simulink model "MCU_CmdTrans"  (R2022b)
settings: Solver=FixedStepDiscrete  StartTime=0.0  StopTime=10.0  FixedStep=0.001  RelTol=1e-3
undefined symbols (not defined in the file or in its folder): ANALOG, cAgeingMode, cCurrentLoopMode, cNoneMode, cParaRecogMode, cSingleBoardMode, cSpeedLoopMode, cTorqueLoopMode, cVvvfOpenMode, FAULT, ParamCfg_CommandSource_u16, ParamCfg_MaxSpeed_u16, ParamCfg_MaxTorque_u16, ParamCfg_Spdouttype_u16, ParamCfg_Vc1Enable_u16, POWER_ON, STANDBY, TESTBED, VEHICLE, WORKING
libraries: simulink x9
(part 1 of 2)
settings Model: DataDictionary=MCU_CmdTrans_Sldd_objects.sldd  Creator=ZYH  LastModifiedBy=ZYH
settings OptimizationCC: DefaultParameterBehavior=Inlined  EnhancedBackFolding=on  PassReuseOutputArgsAs=Individual arguments  OptimizeBlockOrder=speed  DifferentSizesBufferReuse=on  OptimizationCustomize=off  EfficientTunableParamExpr=on
settings DebuggingCC: ParameterTunabilityLossMsg=error
settings SFSimCC: MATLABDynamicMemAlloc=off
settings RTWCC: Description=Embedded Coder  SystemTargetFile=ert.tlc  GenCodeOnly=on  TemplateMakefile=ert_default_tmf
settings CodeAppCC: ForceParamTrailComments=on  IgnoreCustomStorageClasses=off  OperatorAnnotations=on  SimulinkDataObjDesc=on  SFDataObjDesc=on  InsertBlockDesc=on
settings ERTTargetCC: TargetLangStandard=C99 (ISO)  GenerateSampleERTMain=on  InlinedParameterPlacement=NonHierarchical  ERTCustomFileTemplate=example_file_process.tlc

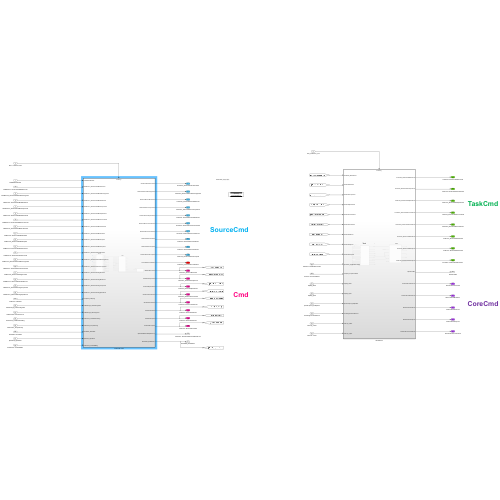
[thumbnail: Simulink's stored preview of the top-level diagram]
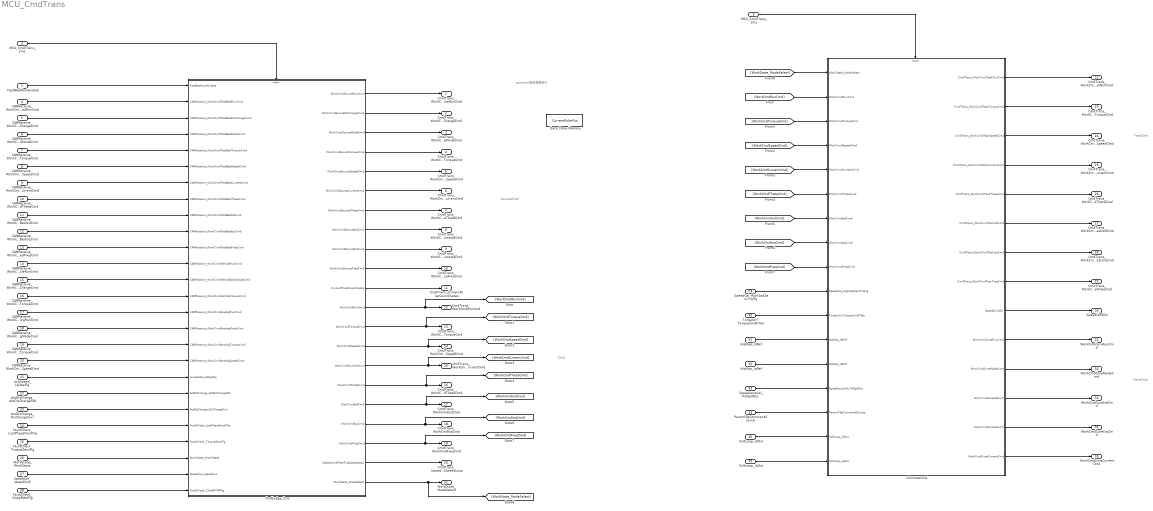
== system MCU_CmdTrans ==
  note: workcmd是否需要简化
  note: TaskCmd
  note: CoreCmd
  note: Cmd
  note: SourceCmd
  TestBedWorkEnable : Inport
  MCU_CmdTrans_1ms : Inport  Port=2  SampleTime=0.001  OutputFunctionCall=on
  MCU_CmdTrans_2ms : Inport  Port=3  SampleTime=0.002  OutputFunctionCall=on
  CANReceive_WorkCmdTestBedRunCmd : Inport  Port=4
  CANReceive_WorkCmdTestBedDisChargeCmd : Inport  Port=5
  CANReceive_WorkCmdTestBedModeCmd : Inport  Port=6
  CANReceive_WorkCmdTestBedTorqueCmd : Inport  Port=7
  CANReceive_WorkCmdTestBedSpeedCmd : Inport  Port=8
  CANReceive_WorkCmdTestBedCurrentCmd : Inport  Port=9
  CANReceive_WorkCmdTestBedThetaCmd : Inport  Port=10
  CANReceive_WorkCmdTestBedIsdCmd : Inport  Port=11
  CANReceive_WorkCmdTestBedIsqCmd : Inport  Port=12
  CANReceive_WorkCmdTestBedFreqCmd : Inport  Port=13
  CANReceive_WorkCmdVehicleRunCmd : Inport  Port=14
  CANReceive_WorkCmdVehicleDisChargeCmd : Inport  Port=15
  CANReceive_WorkCmdVehicleTorqueCmd : Inport  Port=16
  CANReceive_WorkCmdAnalogRunCmd : Inport  Port=17
  CANReceive_WorkCmdAnalogModeCmd : Inport  Port=18
  CANReceive_WorkCmdAnalogTorqueCmd : Inport  Port=19
  CANReceive_WorkCmdAnalogSpeedCmd : Inport  Port=20
  LowSpeed_LsDepFlg : Inport  Port=21
  ActDisCharge_ActDisChargeStd : Inport  Port=22
  ActDisCharge_DisChargeCurr : Inport  Port=23
  FaultCheck_LostPhaseFaultFlg : Inport  Port=24
  FaultCheck_TorqueZeroFlg : Inport  Port=25
  WorkState_WorkState : Inport  Port=26
  SpeedCal_speed2ms : Inport  Port=27
  FaultCheck_ClosePWMFlg : Inport  Port=28
  SpeedCal_HighSpdZeroTrqFlg : Inport  Port=29
  TorqeCtrl_TorqueCmdFilter : Inport  Port=30
  IdqMap_IdRef : Inport  Port=31
  IdqMap_IqRef : Inport  Port=32
  SpeedLoopCal_PidSpdOut : Inport  Port=33
  ParamCfgCommandSource : Inport  Port=34
  VoltLoop_IdOut : Inport  Port=35
  VoltLoop_IqOut : Inport  Port=36
  CmdJudge_2ms : Subsystem
  Data Store Memory : DataStoreMemory  DataStoreName=CurrentPolarFuc  WriteAfterWriteMsg=warning  ShareAcrossModelInstances=on  ShowAdditionalParam=off
  UltimateCmd : Subsystem  TreatAsAtomicUnit=on
  CmdTrans_WorkCmdSourceRunCmd : Outport
  CmdTrans_WorkCmdSourceDisChargeCmd : Outport  Port=2
  CmdTrans_WorkCmdSourceModeCmd : Outport  Port=3
  CmdTrans_WorkCmdSourceTorqueCmd : Outport  Port=4
  CmdTrans_WorkCmdSourceSpeedCmd : Outport  Port=5
  CmdTrans_WorkCmdSourceCurrentCmd : Outport  Port=6
  CmdTrans_WorkCmdSourceThetaCmd : Outport  Port=7
  CmdTrans_WorkCmdSourceIsdCmd : Outport  Port=8
  CmdTrans_WorkCmdSourceIsqCmd : Outport  Port=9
  CmdTrans_WorkCmdSourceFreqCmd : Outport  Port=10
  CmdTrans_CurrentPolarCoordinates : Outport  Port=11
  CmdTrans_WorkCmdRunCmd : Outport  Port=12
  CmdTrans_WorkCmdTorqueCmd : Outport  Port=13
  CmdTrans_WorkCmdSpeedCmd : Outport  Port=14
  CmdTrans_WorkCmdCurrentCmd : Outport  Port=15
  CmdTrans_WorkCmdThetaCmd : Outport  Port=16
  CmdTrans_WorkCmdIsdCmd : Outport  Port=17
  CmdTrans_WorkCmdIsqCmd : Outport  Port=18
  CmdTrans_WorkCmdFreqCmd : Outport  Port=19
  CmdTrans_SpeedCmdFilterFirstSpeedLoop : Outport  Port=20
  WorkState_ModeSelect : Outport  Port=21
  CmdTrans_WorkCmdTaskRunCmd : Outport  Port=22
  CmdTrans_WorkCmdTaskTorqueCmd : Outport  Port=23
  CmdTrans_WorkCmdTaskSpeedCmd : Outport  Port=24
  CmdTrans_WorkCmdTaskCurrentCmd : Outport  Port=25
  CmdTrans_WorkCmdTaskThetaCmd : Outport  Port=26
  CmdTrans_WorkCmdTaskIsdCmd : Outport  Port=27
  CmdTrans_WorkCmdTaskIsqCmd : Outport  Port=28
  CmdTrans_WorkCmdTaskFreqCmd : Outport  Port=29
  SpeedCmdDir : Outport  Port=30
  WorkCmdCoreRunCmd : Outport  Port=31
  WorkCmdCoreModeCmd : Outport  Port=32
  WorkCmdCoreIsdCmd : Outport  Port=33
  WorkCmdCoreIsqCmd : Outport  Port=34
  WorkCmdCoreCurrentCmd : Outport  Port=35
  wires:
  CANReceive_WorkCmdTestBedRunCmd/1 -> CmdJudge_2ms/2(CANReceive_WorkCmdTestBedRunCmd)
  CANReceive_WorkCmdTestBedDisChargeCmd/1 -> CmdJudge_2ms/3(CANReceive_WorkCmdTestBedDisChargeCmd)
  CANReceive_WorkCmdTestBedModeCmd/1 -> CmdJudge_2ms/4(CANReceive_WorkCmdTestBedModeCmd)
  CANReceive_WorkCmdTestBedTorqueCmd/1 -> CmdJudge_2ms/5(CANReceive_WorkCmdTestBedTorqueCmd)
  CANReceive_WorkCmdTestBedSpeedCmd/1 -> CmdJudge_2ms/6(CANReceive_WorkCmdTestBedSpeedCmd)
  CANReceive_WorkCmdTestBedCurrentCmd/1 -> CmdJudge_2ms/7(CANReceive_WorkCmdTestBedCurrentCmd)
  CANReceive_WorkCmdTestBedThetaCmd/1 -> CmdJudge_2ms/8(CANReceive_WorkCmdTestBedThetaCmd)
  CANReceive_WorkCmdTestBedIsdCmd/1 -> CmdJudge_2ms/9(CANReceive_WorkCmdTestBedIsdCmd)
  CANReceive_WorkCmdTestBedIsqCmd/1 -> CmdJudge_2ms/10(CANReceive_WorkCmdTestBedIsqCmd)
  CANReceive_WorkCmdTestBedFreqCmd/1 -> CmdJudge_2ms/11(CANReceive_WorkCmdTestBedFreqCmd)
  CANReceive_WorkCmdVehicleRunCmd/1 -> CmdJudge_2ms/12(CANReceive_WorkCmdVehicleRunCmd)
  CANReceive_WorkCmdVehicleDisChargeCmd/1 -> CmdJudge_2ms/13(CANReceive_WorkCmdVehicleDisChargeCmd)
  CANReceive_WorkCmdVehicleTorqueCmd/1 -> CmdJudge_2ms/14(CANReceive_WorkCmdVehicleTorqueCmd)
  CANReceive_WorkCmdAnalogRunCmd/1 -> CmdJudge_2ms/15(CANReceive_WorkCmdAnalogRunCmd)
  CANReceive_WorkCmdAnalogModeCmd/1 -> CmdJudge_2ms/16(CANReceive_WorkCmdAnalogModeCmd)
  CANReceive_WorkCmdAnalogTorqueCmd/1 -> CmdJudge_2ms/17(CANReceive_WorkCmdAnalogTorqueCmd)
  CANReceive_WorkCmdAnalogSpeedCmd/1 -> CmdJudge_2ms/18(CANReceive_WorkCmdAnalogSpeedCmd)
  MCU_CmdTrans_2ms/1 -> CmdJudge_2ms/Trigger
  TestBedWorkEnable/1 -> CmdJudge_2ms/1(TestBedWorkEnable)
  LowSpeed_LsDepFlg/1 -> CmdJudge_2ms/19(LowSpeed_LsDepFlg)
  ActDisCharge_ActDisChargeStd/1 -> CmdJudge_2ms/20(ActDisCharge_ActDisChargeStd)
  ActDisCharge_DisChargeCurr/1 -> CmdJudge_2ms/21(ActDisCharge_DisChargeCurr)
  FaultCheck_LostPhaseFaultFlg/1 -> CmdJudge_2ms/22(FaultCheck_LostPhaseFaultFlg)
  CmdJudge_2ms/1(WorkCmdSourceRunCmd) -> CmdTrans_WorkCmdSourceRunCmd/1
  CmdJudge_2ms/2(WorkCmdSourceDisChargeCmd) -> CmdTrans_WorkCmdSourceDisChargeCmd/1
  CmdJudge_2ms/3(WorkCmdSourceModeCmd) -> CmdTrans_WorkCmdSourceModeCmd/1
  CmdJudge_2ms/4(WorkCmdSourceTorqueCmd) -> CmdTrans_WorkCmdSourceTorqueCmd/1
  CmdJudge_2ms/5(WorkCmdSourceSpeedCmd) -> CmdTrans_WorkCmdSourceSpeedCmd/1
  CmdJudge_2ms/6(WorkCmdSourceCurrentCmd) -> CmdTrans_WorkCmdSourceCurrentCmd/1
  CmdJudge_2ms/7(WorkCmdSourceThetaCmd) -> CmdTrans_WorkCmdSourceThetaCmd/1
  CmdJudge_2ms/8(WorkCmdSourceIsdCmd) -> CmdTrans_WorkCmdSourceIsdCmd/1
  CmdJudge_2ms/9(WorkCmdSourceIsqCmd) -> CmdTrans_WorkCmdSourceIsqCmd/1
  CmdJudge_2ms/10(WorkCmdSourceFreqCmd) -> CmdTrans_WorkCmdSourceFreqCmd/1
  CmdJudge_2ms/11(CurrentPolarCoordinates) -> CmdTrans_CurrentPolarCoordinates/1
  FaultCheck_TorqueZeroFlg/1 -> CmdJudge_2ms/23(FaultCheck_TorqueZeroFlg)
  WorkState_WorkState/1 -> CmdJudge_2ms/24(WorkState_WorkState)
  SpeedCal_speed2ms/1 -> CmdJudge_2ms/25(SpeedCal_speed2ms)
  FaultCheck_ClosePWMFlg/1 -> CmdJudge_2ms/26(FaultCheck_ClosePWMFlg)
  CmdJudge_2ms/12(WorkCmdRunCmd) -> [WorkCmdRunCmd], CmdTrans_WorkCmdRunCmd/1
  CmdJudge_2ms/13(WorkCmdTorqueCmd) -> [WorkCmdTorqueCmd], CmdTrans_WorkCmdTorqueCmd/1
  CmdJudge_2ms/14(WorkCmdSpeedCmd) -> [WorkCmdSpeedCmd], CmdTrans_WorkCmdSpeedCmd/1
  CmdJudge_2ms/15(WorkCmdCurrentCmd) -> [WorkCmdCurrentCmd], CmdTrans_WorkCmdCurrentCmd/1
  CmdJudge_2ms/16(WorkCmdThetaCmd) -> [WorkCmdThetaCmd], CmdTrans_WorkCmdThetaCmd/1
  CmdJudge_2ms/17(WorkCmdIsdCmd) -> [WorkCmdIsdCmd], CmdTrans_WorkCmdIsdCmd/1
  CmdJudge_2ms/18(WorkCmdIsqCmd) -> [WorkCmdIsqCmd], CmdTrans_WorkCmdIsqCmd/1
  CmdJudge_2ms/19(WorkCmdFreqCmd) -> [WorkCmdFreqCmd], CmdTrans_WorkCmdFreqCmd/1
  CmdJudge_2ms/20(SpeedCmdFilterFirstSpeedLoop) -> CmdTrans_SpeedCmdFilterFirstSpeedLoop/1
  MCU_CmdTrans_1ms/1 -> UltimateCmd/Trigger
  CmdJudge_2ms/21(WorkState_ModeSelect) -> [WorkState_ModeSelect], WorkState_ModeSelect/1
  [WorkState_ModeSelect] -> UltimateCmd/1(WorkState_ModeSelect)
  [WorkCmdRunCmd] -> UltimateCmd/2(WorkCmdRunCmd)
  [WorkCmdTorqueCmd] -> UltimateCmd/3(WorkCmdTorqueCmd)
  [WorkCmdSpeedCmd] -> UltimateCmd/4(WorkCmdSpeedCmd)
  [WorkCmdCurrentCmd] -> UltimateCmd/5(WorkCmdCurrentCmd)
  [WorkCmdThetaCmd] -> UltimateCmd/6(WorkCmdThetaCmd)
  [WorkCmdIsdCmd] -> UltimateCmd/7(WorkCmdIsdCmd)
  [WorkCmdIsqCmd] -> UltimateCmd/8(WorkCmdIsqCmd)
  [WorkCmdFreqCmd] -> UltimateCmd/9(WorkCmdFreqCmd)
  TorqeCtrl_TorqueCmdFilter/1 -> UltimateCmd/11(TorqeCtrl_TorqueCmdFilter)
  SpeedCal_HighSpdZeroTrqFlg/1 -> UltimateCmd/10(SpeedCal_HighSpdZeroTrqFlg)
  UltimateCmd/1(CmdTrans_WorkCmdTaskRunCmd) -> CmdTrans_WorkCmdTaskRunCmd/1
  UltimateCmd/2(CmdTrans_WorkCmdTaskTorqueCmd) -> CmdTrans_WorkCmdTaskTorqueCmd/1
  UltimateCmd/3(CmdTrans_WorkCmdTaskSpeedCmd) -> CmdTrans_WorkCmdTaskSpeedCmd/1
  UltimateCmd/4(CmdTrans_WorkCmdTaskCurrentCmd) -> CmdTrans_WorkCmdTaskCurrentCmd/1
  UltimateCmd/5(CmdTrans_WorkCmdTaskThetaCmd) -> CmdTrans_WorkCmdTaskThetaCmd/1
  UltimateCmd/6(CmdTrans_WorkCmdTaskIsdCmd) -> CmdTrans_WorkCmdTaskIsdCmd/1
  UltimateCmd/7(CmdTrans_WorkCmdTaskIsqCmd) -> CmdTrans_WorkCmdTaskIsqCmd/1
  UltimateCmd/8(CmdTrans_WorkCmdTaskFreqCmd) -> CmdTrans_WorkCmdTaskFreqCmd/1
  UltimateCmd/9(SpeedCmdDir) -> SpeedCmdDir/1
  VoltLoop_IqOut/1 -> UltimateCmd/17(VoltLoop_IqOut)
  IdqMap_IdRef/1 -> UltimateCmd/12(IdqMap_IdRef)
  ParamCfgCommandSource/1 -> UltimateCmd/15(ParamCfgCommandSource)
  VoltLoop_IdOut/1 -> UltimateCmd/16(VoltLoop_IdOut)
  SpeedLoopCal_PidSpdOut/1 -> UltimateCmd/14(SpeedLoopCal_PidSpdOut)
  IdqMap_IqRef/1 -> UltimateCmd/13(IdqMap_IqRef)
  UltimateCmd/10(WorkCmdCoreRunCmd) -> WorkCmdCoreRunCmd/1
  UltimateCmd/11(WorkCmdCoreModeCmd) -> WorkCmdCoreModeCmd/1
  UltimateCmd/12(WorkCmdCoreIsdCmd) -> WorkCmdCoreIsdCmd/1
  UltimateCmd/13(WorkCmdCoreIsqCmd) -> WorkCmdCoreIsqCmd/1
  UltimateCmd/14(WorkCmdCoreCurrentCmd) -> WorkCmdCoreCurrentCmd/1

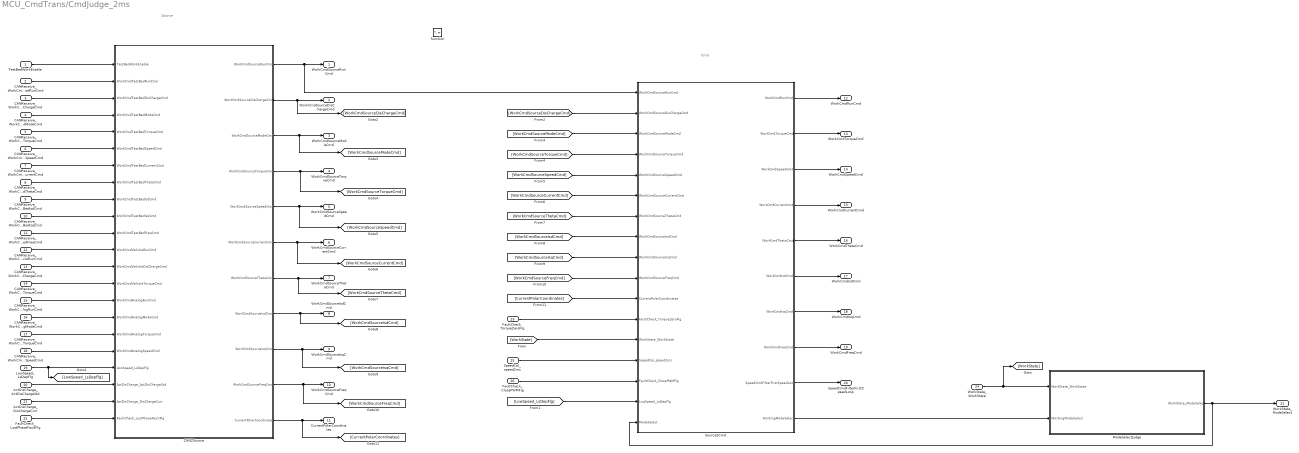
== system MCU_CmdTrans/CmdJudge_2ms ==
  note: Cmd
  note: Source
  TestBedWorkEnable : Inport
  CANReceive_WorkCmdTestBedRunCmd : Inport  Port=2
  CANReceive_WorkCmdTestBedDisChargeCmd : Inport  Port=3
  CANReceive_WorkCmdTestBedModeCmd : Inport  Port=4
  CANReceive_WorkCmdTestBedTorqueCmd : Inport  Port=5
  CANReceive_WorkCmdTestBedSpeedCmd : Inport  Port=6
  CANReceive_WorkCmdTestBedCurrentCmd : Inport  Port=7
  CANReceive_WorkCmdTestBedThetaCmd : Inport  Port=8
  CANReceive_WorkCmdTestBedIsdCmd : Inport  Port=9
  CANReceive_WorkCmdTestBedIsqCmd : Inport  Port=10
  CANReceive_WorkCmdTestBedFreqCmd : Inport  Port=11
  CANReceive_WorkCmdVehicleRunCmd : Inport  Port=12
  CANReceive_WorkCmdVehicleDisChargeCmd : Inport  Port=13
  CANReceive_WorkCmdVehicleTorqueCmd : Inport  Port=14
  CANReceive_WorkCmdAnalogRunCmd : Inport  Port=15
  CANReceive_WorkCmdAnalogModeCmd : Inport  Port=16
  CANReceive_WorkCmdAnalogTorqueCmd : Inport  Port=17
  CANReceive_WorkCmdAnalogSpeedCmd : Inport  Port=18
  LowSpeed_LsDepFlg : Inport  Port=19
  ActDisCharge_ActDisChargeStd : Inport  Port=20
  ActDisCharge_DisChargeCurr : Inport  Port=21
  FaultCheck_LostPhaseFaultFlg : Inport  Port=22
  FaultCheck_TorqueZeroFlg : Inport  Port=23
  WorkState_WorkState : Inport  Port=24
  SpeedCal_speed2ms : Inport  Port=25
  FaultCheck_ClosePWMFlg : Inport  Port=26
  function : TriggerPort  TriggerType=function-call  VariantControl=(inherit)
  CAN2Source : Subsystem  TreatAsAtomicUnit=on
      settings: RTWSystemCode=Nonreusable function
  ModeSelectJudge : Subsystem  TreatAsAtomicUnit=on
      settings: RTWSystemCode=Nonreusable function
  Source2Cmd : Subsystem  TreatAsAtomicUnit=on
      settings: RTWSystemCode=Nonreusable function
  WorkCmdSourceRunCmd : Outport
  WorkCmdSourceDisChargeCmd : Outport  Port=2
  WorkCmdSourceModeCmd : Outport  Port=3
  WorkCmdSourceTorqueCmd : Outport  Port=4
  WorkCmdSourceSpeedCmd : Outport  Port=5
  WorkCmdSourceCurrentCmd : Outport  Port=6
  WorkCmdSourceThetaCmd : Outport  Port=7
  WorkCmdSourceIsdCmd : Outport  Port=8
  WorkCmdSourceIsqCmd : Outport  Port=9
  WorkCmdSourceFreqCmd : Outport  Port=10
  CurrentPolarCoordinates : Outport  Port=11
  WorkCmdRunCmd : Outport  Port=12
  WorkCmdTorqueCmd : Outport  Port=13
  WorkCmdSpeedCmd : Outport  Port=14
  WorkCmdCurrentCmd : Outport  Port=15
  WorkCmdThetaCmd : Outport  Port=16
  WorkCmdIsdCmd : Outport  Port=17
  WorkCmdIsqCmd : Outport  Port=18
  WorkCmdFreqCmd : Outport  Port=19
  SpeedCmdFilterFirstSpeedLoop : Outport  Port=20
  WorkState_ModeSelect : Outport  Port=21
  wires:
  CANReceive_WorkCmdVehicleTorqueCmd/1 -> CAN2Source/14(WorkCmdVehicleTorqueCmd)
  CANReceive_WorkCmdTestBedSpeedCmd/1 -> CAN2Source/6(WorkCmdTestBedSpeedCmd)
  CANReceive_WorkCmdTestBedIsqCmd/1 -> CAN2Source/10(WorkCmdTestBedIsqCmd)
  CANReceive_WorkCmdAnalogModeCmd/1 -> CAN2Source/16(WorkCmdAnalogModeCmd)
  CANReceive_WorkCmdTestBedTorqueCmd/1 -> CAN2Source/5(WorkCmdTestBedTorqueCmd)
  CANReceive_WorkCmdTestBedRunCmd/1 -> CAN2Source/2(WorkCmdTestBedRunCmd)
  CANReceive_WorkCmdTestBedFreqCmd/1 -> CAN2Source/11(WorkCmdTestBedFreqCmd)
  CANReceive_WorkCmdTestBedIsdCmd/1 -> CAN2Source/9(WorkCmdTestBedIsdCmd)
  CANReceive_WorkCmdAnalogRunCmd/1 -> CAN2Source/15(WorkCmdAnalogRunCmd)
  CANReceive_WorkCmdAnalogTorqueCmd/1 -> CAN2Source/17(WorkCmdAnalogTorqueCmd)
  CANReceive_WorkCmdTestBedCurrentCmd/1 -> CAN2Source/7(WorkCmdTestBedCurrentCmd)
  CANReceive_WorkCmdTestBedDisChargeCmd/1 -> CAN2Source/3(WorkCmdTestBedDisChargeCmd)
  CANReceive_WorkCmdVehicleDisChargeCmd/1 -> CAN2Source/13(WorkCmdVehicleDisChargeCmd)
  CANReceive_WorkCmdAnalogSpeedCmd/1 -> CAN2Source/18(WorkCmdAnalogSpeedCmd)
  CANReceive_WorkCmdTestBedThetaCmd/1 -> CAN2Source/8(WorkCmdTestBedThetaCmd)
  CANReceive_WorkCmdTestBedModeCmd/1 -> CAN2Source/4(WorkCmdTestBedModeCmd)
  CANReceive_WorkCmdVehicleRunCmd/1 -> CAN2Source/12(WorkCmdVehicleRunCmd)
  TestBedWorkEnable/1 -> CAN2Source/1(TestBedWorkEnable)
  CAN2Source/11(CurrentPolarCoordinates) -> [CurrentPolarCoordinates], CurrentPolarCoordinates/1
  CAN2Source/2(WorkCmdSourceDisChargeCmd) -> [WorkCmdSourceDisChargeCmd], WorkCmdSourceDisChargeCmd/1
  CAN2Source/3(WorkCmdSourceModeCmd) -> [WorkCmdSourceModeCmd], WorkCmdSourceModeCmd/1
  CAN2Source/4(WorkCmdSourceTorqueCmd) -> [WorkCmdSourceTorqueCmd], WorkCmdSourceTorqueCmd/1
  CAN2Source/5(WorkCmdSourceSpeedCmd) -> [WorkCmdSourceSpeedCmd], WorkCmdSourceSpeedCmd/1
  CAN2Source/6(WorkCmdSourceCurrentCmd) -> [WorkCmdSourceCurrentCmd], WorkCmdSourceCurrentCmd/1
  CAN2Source/7(WorkCmdSourceThetaCmd) -> [WorkCmdSourceThetaCmd], WorkCmdSourceThetaCmd/1
  CAN2Source/8(WorkCmdSourceIsdCmd) -> [WorkCmdSourceIsdCmd], WorkCmdSourceIsdCmd/1
  CAN2Source/9(WorkCmdSourceIsqCmd) -> [WorkCmdSourceIsqCmd], WorkCmdSourceIsqCmd/1
  CAN2Source/10(WorkCmdSourceFreqCmd) -> WorkCmdSourceFreqCmd/1, [WorkCmdSourceFreqCmd]
  LowSpeed_LsDepFlg/1 -> [LowSpeed_LsDepFlg], CAN2Source/19(LowSpeed_LsDepFlg)
  ActDisCharge_DisChargeCurr/1 -> CAN2Source/21(ActDisCharge_DisChargeCurr)
  FaultCheck_LostPhaseFaultFlg/1 -> CAN2Source/22(FaultCheck_LostPhaseFaultFlg)
  ActDisCharge_ActDisChargeStd/1 -> CAN2Source/20(ActDisCharge_ActDisChargeStd)
  ModeSelectJudge/1(WorkState_ModeSelect) -> WorkState_ModeSelect/1, Source2Cmd/17(ModeSelect)
  FaultCheck_TorqueZeroFlg/1 -> Source2Cmd/12(FaultCheck_TorqueZeroFlg)
  SpeedCal_speed2ms/1 -> Source2Cmd/14(SpeedCal_speed2ms)
  WorkState_WorkState/1 -> [WorkState], ModeSelectJudge/1(WorkState_WorkState)
  FaultCheck_ClosePWMFlg/1 -> Source2Cmd/15(FaultCheck_ClosePWMFlg)
  Source2Cmd/1(WorkCmdRunCmd) -> WorkCmdRunCmd/1
  Source2Cmd/2(WorkCmdTorqueCmd) -> WorkCmdTorqueCmd/1
  Source2Cmd/3(WorkCmdSpeedCmd) -> WorkCmdSpeedCmd/1
  Source2Cmd/4(WorkCmdCurrentCmd) -> WorkCmdCurrentCmd/1
  Source2Cmd/5(WorkCmdThetaCmd) -> WorkCmdThetaCmd/1
  Source2Cmd/6(WorkCmdIsdCmd) -> WorkCmdIsdCmd/1
  Source2Cmd/7(WorkCmdIsqCmd) -> WorkCmdIsqCmd/1
  Source2Cmd/8(WorkCmdFreqCmd) -> WorkCmdFreqCmd/1
  Source2Cmd/9(SpeedCmdFilterFirstSpeedLoop) -> SpeedCmdFilterFirstSpeedLoop/1
  CAN2Source/1(WorkCmdSourceRunCmd) -> Source2Cmd/1(WorkCmdSourceRunCmd), WorkCmdSourceRunCmd/1
  [WorkCmdSourceDisChargeCmd] -> Source2Cmd/2(WorkCmdSourceDisChargeCmd)
  [WorkCmdSourceFreqCmd] -> Source2Cmd/10(WorkCmdSourceFreqCmd)
  [WorkCmdSourceModeCmd] -> Source2Cmd/3(WorkCmdSourceModeCmd)
  [WorkCmdSourceTorqueCmd] -> Source2Cmd/4(WorkCmdSourceTorqueCmd)
  [WorkCmdSourceSpeedCmd] -> Source2Cmd/5(WorkCmdSourceSpeedCmd)
  [WorkCmdSourceCurrentCmd] -> Source2Cmd/6(WorkCmdSourceCurrentCmd)
  [WorkCmdSourceThetaCmd] -> Source2Cmd/7(WorkCmdSourceThetaCmd)
  [WorkCmdSourceIsdCmd] -> Source2Cmd/8(WorkCmdSourceIsdCmd)
  [WorkCmdSourceIsqCmd] -> Source2Cmd/9(WorkCmdSourceIsqCmd)
  [CurrentPolarCoordinates] -> Source2Cmd/11(CurrentPolarCoordinates)
  [WorkState] -> Source2Cmd/13(WorkState_WorkState)
  Source2Cmd/10(WorkingModeSelect) -> ModeSelectJudge/2(WorkingModeSelect)
  [LowSpeed_LsDepFlg] -> Source2Cmd/16(LowSpeed_LsDepFlg)

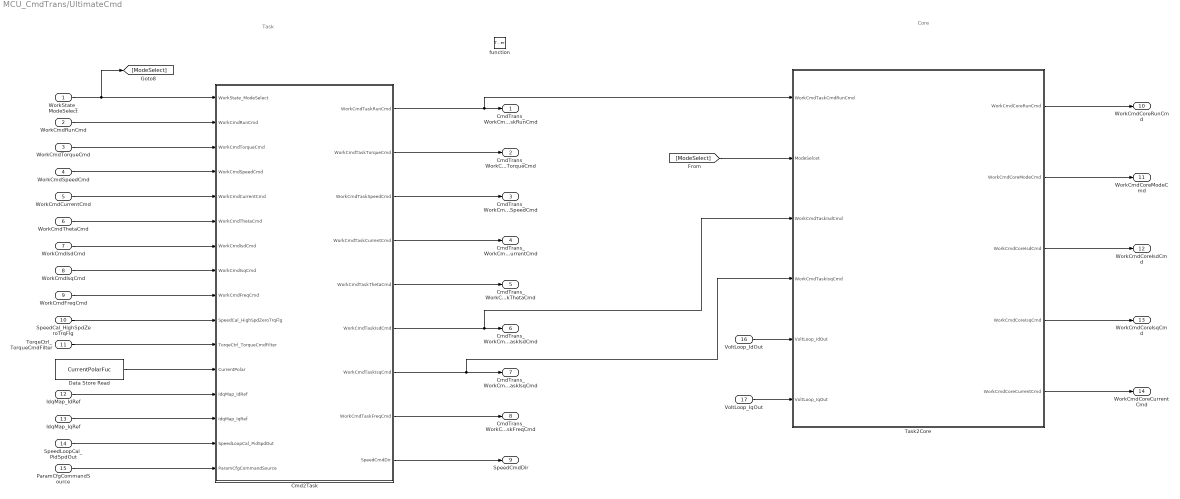
== system MCU_CmdTrans/UltimateCmd ==
  note: Core
  note: Task
  WorkState_ModeSelect : Inport
  WorkCmdRunCmd : Inport  Port=2
  WorkCmdTorqueCmd : Inport  Port=3
  WorkCmdSpeedCmd : Inport  Port=4
  WorkCmdCurrentCmd : Inport  Port=5
  WorkCmdThetaCmd : Inport  Port=6
  WorkCmdIsdCmd : Inport  Port=7
  WorkCmdIsqCmd : Inport  Port=8
  WorkCmdFreqCmd : Inport  Port=9
  SpeedCal_HighSpdZeroTrqFlg : Inport  Port=10
  TorqeCtrl_TorqueCmdFilter : Inport  Port=11
  IdqMap_IdRef : Inport  Port=12
  IdqMap_IqRef : Inport  Port=13
  SpeedLoopCal_PidSpdOut : Inport  Port=14
  ParamCfgCommandSource : Inport  Port=15
  VoltLoop_IdOut : Inport  Port=16
  VoltLoop_IqOut : Inport  Port=17
  function : TriggerPort  TriggerType=function-call  VariantControl=(inherit)
  Cmd2Task : Subsystem
  Data Store Read : DataStoreRead  DataStoreName=CurrentPolarFuc  IndexOptions=Index vector (dialog)  Indices=1  OutputSizes=1
  Task2Core : Subsystem
  CmdTrans_WorkCmdTaskRunCmd : Outport
  CmdTrans_WorkCmdTaskTorqueCmd : Outport  Port=2
  CmdTrans_WorkCmdTaskSpeedCmd : Outport  Port=3
  CmdTrans_WorkCmdTaskCurrentCmd : Outport  Port=4
  CmdTrans_WorkCmdTaskThetaCmd : Outport  Port=5
  CmdTrans_WorkCmdTaskIsdCmd : Outport  Port=6
  CmdTrans_WorkCmdTaskIsqCmd : Outport  Port=7
  CmdTrans_WorkCmdTaskFreqCmd : Outport  Port=8
  SpeedCmdDir : Outport  Port=9
  WorkCmdCoreRunCmd : Outport  Port=10
  WorkCmdCoreModeCmd : Outport  Port=11
  WorkCmdCoreIsdCmd : Outport  Port=12
  WorkCmdCoreIsqCmd : Outport  Port=13
  WorkCmdCoreCurrentCmd : Outport  Port=14
  wires:
  WorkState_ModeSelect/1 -> [ModeSelect], Cmd2Task/1(WorkState_ModeSelect)
  WorkCmdRunCmd/1 -> Cmd2Task/2(WorkCmdRunCmd)
  WorkCmdTorqueCmd/1 -> Cmd2Task/3(WorkCmdTorqueCmd)
  WorkCmdSpeedCmd/1 -> Cmd2Task/4(WorkCmdSpeedCmd)
  WorkCmdCurrentCmd/1 -> Cmd2Task/5(WorkCmdCurrentCmd)
  WorkCmdThetaCmd/1 -> Cmd2Task/6(WorkCmdThetaCmd)
  WorkCmdIsdCmd/1 -> Cmd2Task/7(WorkCmdIsdCmd)
  WorkCmdIsqCmd/1 -> Cmd2Task/8(WorkCmdIsqCmd)
  WorkCmdFreqCmd/1 -> Cmd2Task/9(WorkCmdFreqCmd)
  SpeedCal_HighSpdZeroTrqFlg/1 -> Cmd2Task/10(SpeedCal_HighSpdZeroTrqFlg)
  TorqeCtrl_TorqueCmdFilter/1 -> Cmd2Task/11(TorqeCtrl_TorqueCmdFilter)
  Data Store Read/1 -> Cmd2Task/12(CurrentPolar)
  Cmd2Task/1(WorkCmdTaskRunCmd) -> Task2Core/1(WorkCmdTaskCmdRunCmd), CmdTrans_WorkCmdTaskRunCmd/1
  Cmd2Task/2(WorkCmdTaskTorqueCmd) -> CmdTrans_WorkCmdTaskTorqueCmd/1
  Cmd2Task/3(WorkCmdTaskSpeedCmd) -> CmdTrans_WorkCmdTaskSpeedCmd/1
  Cmd2Task/4(WorkCmdTaskCurrentCmd) -> CmdTrans_WorkCmdTaskCurrentCmd/1
  Cmd2Task/5(WorkCmdTaskThetaCmd) -> CmdTrans_WorkCmdTaskThetaCmd/1
  Cmd2Task/7(WorkCmdTaskIsqCmd) -> Task2Core/4(WorkCmdTaskIsqCmd), CmdTrans_WorkCmdTaskIsqCmd/1
  Cmd2Task/8(WorkCmdTaskFreqCmd) -> CmdTrans_WorkCmdTaskFreqCmd/1
  Cmd2Task/9(SpeedCmdDir) -> SpeedCmdDir/1
  [ModeSelect] -> Task2Core/2(ModeSelcet)
  IdqMap_IqRef/1 -> Cmd2Task/14(IdqMap_IqRef)
  SpeedLoopCal_PidSpdOut/1 -> Cmd2Task/15(SpeedLoopCal_PidSpdOut)
  IdqMap_IdRef/1 -> Cmd2Task/13(IdqMap_IdRef)
  ParamCfgCommandSource/1 -> Cmd2Task/16(ParamCfgCommandSource)
  Cmd2Task/6(WorkCmdTaskIsdCmd) -> Task2Core/3(WorkCmdTaskIsdCmd), CmdTrans_WorkCmdTaskIsdCmd/1
  VoltLoop_IdOut/1 -> Task2Core/5(VoltLoop_IdOut)
  VoltLoop_IqOut/1 -> Task2Core/6(VoltLoop_IqOut)
  Task2Core/1(WorkCmdCoreRunCmd) -> WorkCmdCoreRunCmd/1
  Task2Core/3(WorkCmdCoreIsdCmd) -> WorkCmdCoreIsdCmd/1
  Task2Core/2(WorkCmdCoreModeCmd) -> WorkCmdCoreModeCmd/1
  Task2Core/4(WorkCmdCoreIsqCmd) -> WorkCmdCoreIsqCmd/1
  Task2Core/5(WorkCmdCoreCurrentCmd) -> WorkCmdCoreCurrentCmd/1

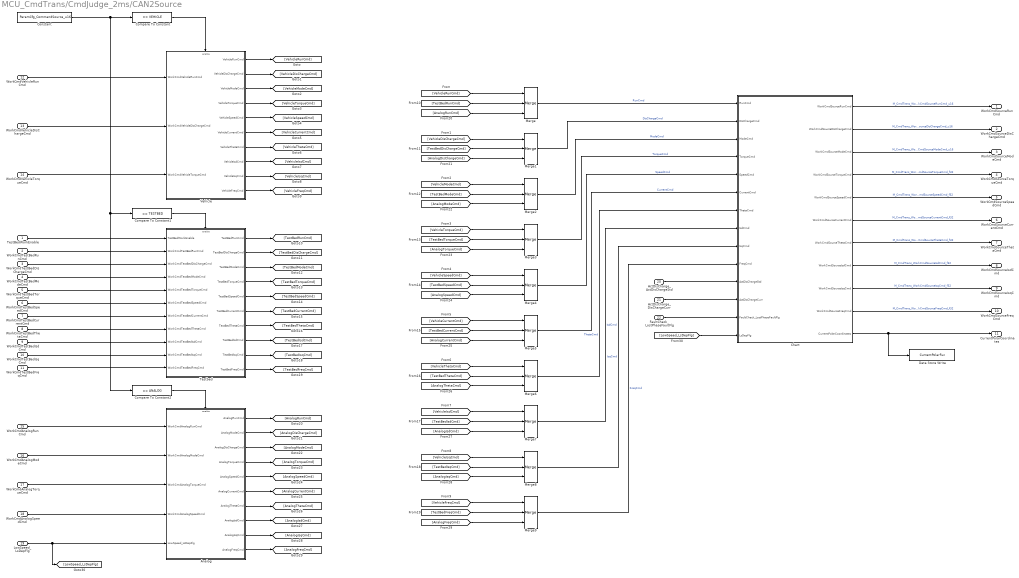
== system MCU_CmdTrans/CmdJudge_2ms/CAN2Source ==
  TestBedWorkEnable : Inport
  WorkCmdTestBedRunCmd : Inport  Port=2
  WorkCmdTestBedDisChargeCmd : Inport  Port=3
  WorkCmdTestBedModeCmd : Inport  Port=4
  WorkCmdTestBedTorqueCmd : Inport  Port=5
  WorkCmdTestBedSpeedCmd : Inport  Port=6
  WorkCmdTestBedCurrentCmd : Inport  Port=7
  WorkCmdTestBedThetaCmd : Inport  Port=8
  WorkCmdTestBedIsdCmd : Inport  Port=9
  WorkCmdTestBedIsqCmd : Inport  Port=10
  WorkCmdTestBedFreqCmd : Inport  Port=11
  WorkCmdVehicleRunCmd : Inport  Port=12
  WorkCmdVehicleDisChargeCmd : Inport  Port=13
  WorkCmdVehicleTorqueCmd : Inport  Port=14
  WorkCmdAnalogRunCmd : Inport  Port=15
  WorkCmdAnalogModeCmd : Inport  Port=16
  WorkCmdAnalogTorqueCmd : Inport  Port=17
  WorkCmdAnalogSpeedCmd : Inport  Port=18
  LowSpeed_LsDepFlg : Inport  Port=19
  ActDisCharge_ActDisChargeStd : Inport  Port=20
  ActDisCharge_DisChargeCurr : Inport  Port=21
  FaultCheck_LostPhaseFaultFlg : Inport  Port=22
  Analog : Subsystem  TreatAsAtomicUnit=on
  Chart : Stateflow chart  TreatAsAtomicUnit=on
  Compare To Constant : simulink/Logic and Bit Operations/Compare To Constant  relop===  const=VEHICLE  OutDataTypeStr=boolean
  Compare To Constant1 : simulink/Logic and Bit Operations/Compare To Constant  relop===  const=TESTBED  OutDataTypeStr=boolean
  Compare To Constant2 : simulink/Logic and Bit Operations/Compare To Constant  relop===  const=ANALOG  OutDataTypeStr=boolean
  Constant : Constant  Value=ParamCfg_CommandSource_u16
  Data Store Write : DataStoreWrite  DataStoreName=CurrentPolarFuc  IndexOptions=Index vector (dialog)  Indices=1  OutputSizes=1
  Merge{,1..9} (10 alike) : Merge  Inputs=3
  Testbed : Subsystem  TreatAsAtomicUnit=on
  Vehicle : Subsystem
  WorkCmdSourceRunCmd : Outport
  WorkCmdSourceDisChargeCmd : Outport  Port=2
  WorkCmdSourceModeCmd : Outport  Port=3
  WorkCmdSourceTorqueCmd : Outport  Port=4
  WorkCmdSourceSpeedCmd : Outport  Port=5
  WorkCmdSourceCurrentCmd : Outport  Port=6
  WorkCmdSourceThetaCmd : Outport  Port=7
  WorkCmdSourceIsdCmd : Outport  Port=8
  WorkCmdSourceIsqCmd : Outport  Port=9
  WorkCmdSourceFreqCmd : Outport  Port=10
  CurrentPolarCoordinates : Outport  Port=11
  wires:
  Constant/1 -> Compare To Constant2/1, Compare To Constant1/1, Compare To Constant/1
  Compare To Constant/1 -> Vehicle/Enable
  WorkCmdVehicleRunCmd/1 -> Vehicle/1(WorkCmdVehicleRunCmd)
  WorkCmdVehicleDisChargeCmd/1 -> Vehicle/2(WorkCmdVehicleDisChargeCmd)
  WorkCmdVehicleTorqueCmd/1 -> Vehicle/3(WorkCmdVehicleTorqueCmd)
  Compare To Constant1/1 -> Testbed/Enable
  WorkCmdTestBedModeCmd/1 -> Testbed/4(WorkCmdTestBedModeCmd)
  WorkCmdTestBedTorqueCmd/1 -> Testbed/5(WorkCmdTestBedTorqueCmd)
  WorkCmdTestBedDisChargeCmd/1 -> Testbed/3(WorkCmdTestBedDisChargeCmd)
  WorkCmdTestBedSpeedCmd/1 -> Testbed/6(WorkCmdTestBedSpeedCmd)
  WorkCmdTestBedRunCmd/1 -> Testbed/2(WorkCmdTestBedRunCmd)
  WorkCmdTestBedCurrentCmd/1 -> Testbed/7(WorkCmdTestBedCurrentCmd)
  WorkCmdTestBedThetaCmd/1 -> Testbed/8(WorkCmdTestBedThetaCmd)
  WorkCmdTestBedIsdCmd/1 -> Testbed/9(WorkCmdTestBedIsdCmd)
  WorkCmdTestBedIsqCmd/1 -> Testbed/10(WorkCmdTestBedIsqCmd)
  WorkCmdTestBedFreqCmd/1 -> Testbed/11(WorkCmdTestBedFreqCmd)
  Compare To Constant2/1 -> Analog/Enable
  WorkCmdAnalogRunCmd/1 -> Analog/1(WorkCmdAnalogRunCmd)
  WorkCmdAnalogModeCmd/1 -> Analog/2(WorkCmdAnalogModeCmd)
  WorkCmdAnalogTorqueCmd/1 -> Analog/3(WorkCmdAnalogTorqueCmd)
  WorkCmdAnalogSpeedCmd/1 -> Analog/4(WorkCmdAnalogSpeedCmd)
  TestBedWorkEnable/1 -> Testbed/1(TestBedWorkEnable)
  Vehicle/1(VehicleRunCmd) -> [VehicleRunCmd]
  Vehicle/2(VehicleDisChargeCmd) -> [VehicleDisChargeCmd]
  Vehicle/3(VehicleModeCmd) -> [VehicleModeCmd]
  Vehicle/4(VehicleTorqueCmd) -> [VehicleTorqueCmd]
  Vehicle/5(VehicleSpeedCmd) -> [VehicleSpeedCmd]
  Vehicle/6(VehicleCurrentCmd) -> [VehicleCurrentCmd]
  Vehicle/7(VehicleThetaCmd) -> [VehicleThetaCmd]
  Vehicle/8(VehicleIsdCmd) -> [VehicleIsdCmd]
  Vehicle/9(VehicleIsqCmd) -> [VehicleIsqCmd]
  Vehicle/10(VehicleFreqCmd) -> [VehicleFreqCmd]
  Testbed/2(TestBedDisChargeCmd) -> [TestBedDisChargeCmd]
  Testbed/3(TestBedModeCmd) -> [TestBedModeCmd]
  Testbed/4(TestBedTorqueCmd) -> [TestBedTorqueCmd]
  Testbed/5(TestBedSpeedCmd) -> [TestBedSpeedCmd]
  Testbed/6(TestBedCurrentCmd) -> [TestBedCurrentCmd]
  Testbed/7(TestBedThetaCmd) -> [TestBedThetaCmd]
  Testbed/8(TestBedIsdCmd) -> [TestBedIsdCmd]
  Testbed/9(TestBedIsqCmd) -> [TestBedIsqCmd]
  Testbed/10(TestBedFreqCmd) -> [TestBedFreqCmd]
  Testbed/1(TestBedRunCmd) -> [TestBedRunCmd]
  Analog/2(AnalogModeCmd) -> [AnalogDisChargeCmd]
  Analog/3(AnalogDisChargeCmd) -> [AnalogModeCmd]
  Analog/4(AnalogTorqueCmd) -> [AnalogTorqueCmd]
  Analog/5(AnalogSpeedCmd) -> [AnalogSpeedCmd]
  Analog/6(AnalogCurrentCmd) -> [AnalogCurrentCmd]
  Analog/7(AnalogThetaCmd) -> [AnalogThetaCmd]
  Analog/8(AnalogIsdCmd) -> [AnalogIsdCmd]
  Analog/9(AnalogIsqCmd) -> [AnalogIsqCmd]
  Analog/10(AnalogFreqCmd) -> [AnalogFreqCmd]
  Analog/1(AnalogRunCmd) -> [AnalogRunCmd]
  [VehicleRunCmd] -> Merge/1
  [VehicleDisChargeCmd] -> Merge1/1
  [VehicleModeCmd] -> Merge2/1
  [VehicleTorqueCmd] -> Merge3/1
  [VehicleSpeedCmd] -> Merge4/1
  [VehicleFreqCmd] -> Merge9/1
  [VehicleCurrentCmd] -> Merge5/1
  [VehicleThetaCmd] -> Merge6/1
  [VehicleIsdCmd] -> Merge7/1
  [VehicleIsqCmd] -> Merge8/1
  [TestBedRunCmd] -> Merge/2
  [TestBedDisChargeCmd] -> Merge1/2
  [TestBedModeCmd] -> Merge2/2
  [TestBedTorqueCmd] -> Merge3/2
  [TestBedSpeedCmd] -> Merge4/2
  [TestBedCurrentCmd] -> Merge5/2
  [TestBedThetaCmd] -> Merge6/2
  [TestBedIsdCmd] -> Merge7/2
  [TestBedIsqCmd] -> Merge8/2
  [TestBedFreqCmd] -> Merge9/2
  [AnalogFreqCmd] -> Merge9/3
  [AnalogRunCmd] -> Merge/3
  [AnalogDisChargeCmd] -> Merge1/3
  [AnalogModeCmd] -> Merge2/3
  [AnalogTorqueCmd] -> Merge3/3
  [AnalogSpeedCmd] -> Merge4/3
  [AnalogCurrentCmd] -> Merge5/3
  [AnalogThetaCmd] -> Merge6/3
  [AnalogIsdCmd] -> Merge7/3
  [AnalogIsqCmd] -> Merge8/3
  Merge/1 -> Chart/1(RunCmd)  "RunCmd"
  Merge1/1 -> Chart/2(DisChargeCmd)  "DisChargeCmd"
  Merge2/1 -> Chart/3(ModeCmd)  "ModeCmd"
  Merge3/1 -> Chart/4(TorqueCmd)  "TorqueCmd"
  Merge4/1 -> Chart/5(SpeedCmd)  "SpeedCmd"
  Merge5/1 -> Chart/6(CurrentCmd)  "CurrentCmd"
  Merge6/1 -> Chart/7(ThetaCmd)  "ThetaCmd"
  Merge7/1 -> Chart/8(IsdCmd)  "IsdCmd"
  Merge8/1 -> Chart/9(IsqCmd)  "IsqCmd"
  Merge9/1 -> Chart/10(FreqCmd)  "FreqCmd"
  LowSpeed_LsDepFlg/1 -> [LowSpeed_LsDepFlg], Analog/5(LowSpeed_LsDepFlg)
  Chart/1(WorkCmdSourceRunCmd) -> WorkCmdSourceRunCmd/1  "M_CmdTrans_WorkCmdSourceRunCmd_u16"
  Chart/2(WorkCmdSourceDisChargeCmd) -> WorkCmdSourceDisChargeCmd/1  "M_CmdTrans_WorkCmdSourceDisChargeCmd_u16"
  Chart/3(WorkCmdSourceModeCmd) -> WorkCmdSourceModeCmd/1  "M_CmdTrans_WorkCmdSourceModeCmd_u16"
  Chart/4(WorkCmdSourceTorqueCmd) -> WorkCmdSourceTorqueCmd/1  "M_CmdTrans_WorkCmdSourceTorqueCmd_f32"
  Chart/5(WorkCmdSourceSpeedCmd) -> WorkCmdSourceSpeedCmd/1  "M_CmdTrans_WorkCmdSourceSpeedCmd_f32"
  Chart/6(WorkCmdSourceCurrentCmd) -> WorkCmdSourceCurrentCmd/1  "M_CmdTrans_WorkCmdSourceCurrentCmd_f32"
  Chart/7(WorkCmdSourceThetaCmd) -> WorkCmdSourceThetaCmd/1  "M_CmdTrans_WorkCmdSourceThetaCmd_f32"
  Chart/8(WorkCmdSourceIsdCmd) -> WorkCmdSourceIsdCmd/1  "M_CmdTrans_WorkCmdSourceIsdCmd_f32"
  Chart/9(WorkCmdSourceIsqCmd) -> WorkCmdSourceIsqCmd/1  "M_CmdTrans_WorkCmdSourceIsqCmd_f32"
  Chart/10(WorkCmdSourceFreqCmd) -> WorkCmdSourceFreqCmd/1  "M_CmdTrans_WorkCmdSourceFreqCmd_f32"
  ActDisCharge_ActDisChargeStd/1 -> Chart/11(ActDisChargeStd)
  ActDisCharge_DisChargeCurr/1 -> Chart/12(ActDisChargeCurr)
  FaultCheck_LostPhaseFaultFlg/1 -> Chart/13(FaultCheck_LostPhaseFaultFlg)
  [LowSpeed_LsDepFlg] -> Chart/14(LsDepFlg)
  Chart/11(CurrentPolarCoordinates) -> Data Store Write/1, CurrentPolarCoordinates/1

== system MCU_CmdTrans/CmdJudge_2ms/ModeSelectJudge ==
  WorkState_WorkState : Inport
  WorkingModeSelect : Inport  Port=2
  Compare To Constant : simulink/Logic and Bit Operations/Compare To Constant  relop===  const=FAULT  OutDataTypeStr=boolean
  Compare To Constant1 : simulink/Logic and Bit Operations/Compare To Constant  relop===  const=POWER_ON  OutDataTypeStr=boolean
  Compare To Constant2 : simulink/Logic and Bit Operations/Compare To Constant  relop===  const=STANDBY  OutDataTypeStr=boolean
  Constant1 : Constant  Value=cNoneMode  VectorParams1D=off  OutDataTypeStr=uint16
  Logical Operator : Logic  Operator=OR  Inputs=3  AllPortsSameDT=off  OutDataTypeStr=boolean
  Switch : Switch  Criteria=u2 ~= 0  SaturateOnIntegerOverflow=off  InputSameDT=off
  WorkState_ModeSelect : Outport
  wires:
  Constant1/1 -> Switch/1
  Compare To Constant/1 -> Logical Operator/1
  Logical Operator/1 -> Switch/2
  WorkState_WorkState/1 -> Compare To Constant2/1, Compare To Constant1/1, Compare To Constant/1
  Compare To Constant2/1 -> Logical Operator/3
  Compare To Constant1/1 -> Logical Operator/2
  WorkingModeSelect/1 -> Switch/3
  Switch/1 -> WorkState_ModeSelect/1

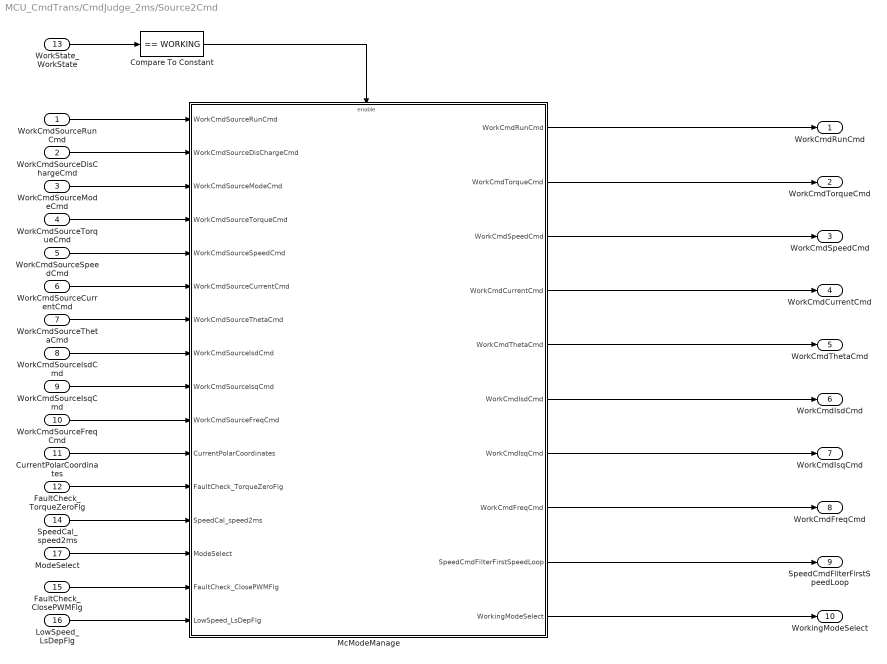
== system MCU_CmdTrans/CmdJudge_2ms/Source2Cmd ==
  WorkCmdSourceRunCmd : Inport
  WorkCmdSourceDisChargeCmd : Inport  Port=2
  WorkCmdSourceModeCmd : Inport  Port=3
  WorkCmdSourceTorqueCmd : Inport  Port=4
  WorkCmdSourceSpeedCmd : Inport  Port=5
  WorkCmdSourceCurrentCmd : Inport  Port=6
  WorkCmdSourceThetaCmd : Inport  Port=7
  WorkCmdSourceIsdCmd : Inport  Port=8
  WorkCmdSourceIsqCmd : Inport  Port=9
  WorkCmdSourceFreqCmd : Inport  Port=10
  CurrentPolarCoordinates : Inport  Port=11
  FaultCheck_TorqueZeroFlg : Inport  Port=12
  WorkState_WorkState : Inport  Port=13
  SpeedCal_speed2ms : Inport  Port=14
  FaultCheck_ClosePWMFlg : Inport  Port=15
  LowSpeed_LsDepFlg : Inport  Port=16
  ModeSelect : Inport  Port=17
  Compare To Constant : simulink/Logic and Bit Operations/Compare To Constant  relop===  const=WORKING  OutDataTypeStr=boolean
  McModeManage : Subsystem  TreatAsAtomicUnit=on
  WorkCmdRunCmd : Outport
  WorkCmdTorqueCmd : Outport  Port=2
  WorkCmdSpeedCmd : Outport  Port=3
  WorkCmdCurrentCmd : Outport  Port=4
  WorkCmdThetaCmd : Outport  Port=5
  WorkCmdIsdCmd : Outport  Port=6
  WorkCmdIsqCmd : Outport  Port=7
  WorkCmdFreqCmd : Outport  Port=8
  SpeedCmdFilterFirstSpeedLoop : Outport  Port=9
  WorkingModeSelect : Outport  Port=10
  wires:
  WorkState_WorkState/1 -> Compare To Constant/1
  Compare To Constant/1 -> McModeManage/Enable
  WorkCmdSourceDisChargeCmd/1 -> McModeManage/2(WorkCmdSourceDisChargeCmd)
  WorkCmdSourceRunCmd/1 -> McModeManage/1(WorkCmdSourceRunCmd)
  WorkCmdSourceModeCmd/1 -> McModeManage/3(WorkCmdSourceModeCmd)
  WorkCmdSourceTorqueCmd/1 -> McModeManage/4(WorkCmdSourceTorqueCmd)
  WorkCmdSourceSpeedCmd/1 -> McModeManage/5(WorkCmdSourceSpeedCmd)
  WorkCmdSourceCurrentCmd/1 -> McModeManage/6(WorkCmdSourceCurrentCmd)
  WorkCmdSourceThetaCmd/1 -> McModeManage/7(WorkCmdSourceThetaCmd)
  WorkCmdSourceIsdCmd/1 -> McModeManage/8(WorkCmdSourceIsdCmd)
  WorkCmdSourceIsqCmd/1 -> McModeManage/9(WorkCmdSourceIsqCmd)
  WorkCmdSourceFreqCmd/1 -> McModeManage/10(WorkCmdSourceFreqCmd)
  CurrentPolarCoordinates/1 -> McModeManage/11(CurrentPolarCoordinates)
  ModeSelect/1 -> McModeManage/14(ModeSelect)
  FaultCheck_TorqueZeroFlg/1 -> McModeManage/12(FaultCheck_TorqueZeroFlg)
  SpeedCal_speed2ms/1 -> McModeManage/13(SpeedCal_speed2ms)
  FaultCheck_ClosePWMFlg/1 -> McModeManage/15(FaultCheck_ClosePWMFlg)
  McModeManage/1(WorkCmdRunCmd) -> WorkCmdRunCmd/1
  McModeManage/9(SpeedCmdFilterFirstSpeedLoop) -> SpeedCmdFilterFirstSpeedLoop/1
  McModeManage/2(WorkCmdTorqueCmd) -> WorkCmdTorqueCmd/1
  McModeManage/3(WorkCmdSpeedCmd) -> WorkCmdSpeedCmd/1
  McModeManage/4(WorkCmdCurrentCmd) -> WorkCmdCurrentCmd/1
  McModeManage/5(WorkCmdThetaCmd) -> WorkCmdThetaCmd/1
  McModeManage/6(WorkCmdIsdCmd) -> WorkCmdIsdCmd/1
  McModeManage/7(WorkCmdIsqCmd) -> WorkCmdIsqCmd/1
  McModeManage/8(WorkCmdFreqCmd) -> WorkCmdFreqCmd/1
  McModeManage/10(WorkingModeSelect) -> WorkingModeSelect/1
  LowSpeed_LsDepFlg/1 -> McModeManage/16(LowSpeed_LsDepFlg)

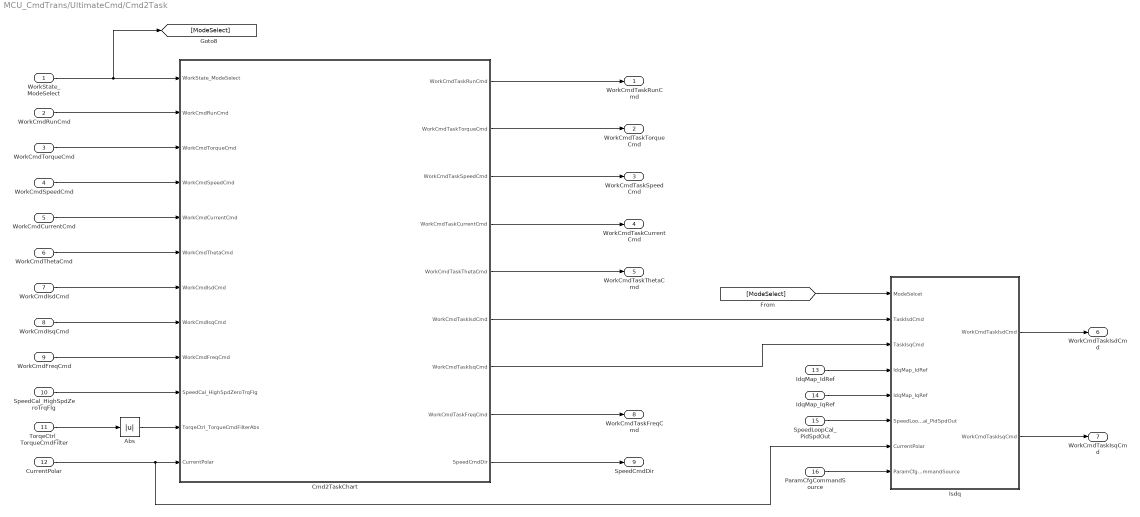
== system MCU_CmdTrans/UltimateCmd/Cmd2Task ==
  WorkState_ModeSelect : Inport
  WorkCmdRunCmd : Inport  Port=2
  WorkCmdTorqueCmd : Inport  Port=3
  WorkCmdSpeedCmd : Inport  Port=4
  WorkCmdCurrentCmd : Inport  Port=5
  WorkCmdThetaCmd : Inport  Port=6
  WorkCmdIsdCmd : Inport  Port=7
  WorkCmdIsqCmd : Inport  Port=8
  WorkCmdFreqCmd : Inport  Port=9
  SpeedCal_HighSpdZeroTrqFlg : Inport  Port=10
  TorqeCtrl_TorqueCmdFilter : Inport  Port=11
  CurrentPolar : Inport  Port=12
  IdqMap_IdRef : Inport  Port=13
  IdqMap_IqRef : Inport  Port=14
  SpeedLoopCal_PidSpdOut : Inport  Port=15
  ParamCfgCommandSource : Inport  Port=16
  Abs : Abs  SaturateOnIntegerOverflow=off
  Cmd2TaskChart : Stateflow chart  TreatAsAtomicUnit=on
      settings: PortSchema="{\"entries\":[{\"content\":{\"sides\":[{\"content\":{\"connectorIds\":[\"In2\",\"In3\",\"In4\",\"In5\",\"In6\",\"In7\",\"In1\",\"In8\",\"In9\",\"In10\",\"In11\",\"In12\"]},\"type\":\"ConnectorPlacement.EquallySpacedRectSide\",\"uuid\":\"3aeab0a9-977f-4d7e-9da7-61fabe5cb386\"},{\"content\":{\"connectorIds\":[\"Out1\",\"Out2\",\"Out3\",\"Out4\",\"Out5\",\"Out6\",\"Out7\",\"Out8\",\"Out9\"],\"side\":\"RIGHT\"},\"type\":\"ConnectorPlacement.EquallySpacedRectSide\",\"uuid\":\"52d65e32-3a7d-4d72-b988-d1b9ef3f3299\"},{\"content\":{\"connectorIds\":[],\"side\":\"TOP\"},\"type\":\"ConnectorPlacement.EquallySpacedRectSide\",\"uuid\":\"7eee4f92-79ee-4dfc-b51c-d644466ec602\"},{\"content\":{\"connectorIds\":[],\"side\":\"BOTTOM\"},\"type\":\"ConnectorPlacement.EquallySpacedRectSide\",\"uuid\":\"a847cf42-6c44-46d8-9270-33361270c7f2\"}]},\"type\":\"ConnectorPlacement.EquallySpacedConnector\",\"uuid\":\"d7c8bde0-45fa-4435-a641-175901423035\"}],\"packageUris\":[\"http://schema.mathworks.com/mf0/Connector/R2020b\"],\"version\":\"1.0\"}"
  Isdq : Subsystem
  WorkCmdTaskRunCmd : Outport
  WorkCmdTaskTorqueCmd : Outport  Port=2
  WorkCmdTaskSpeedCmd : Outport  Port=3
  WorkCmdTaskCurrentCmd : Outport  Port=4
  WorkCmdTaskThetaCmd : Outport  Port=5
  WorkCmdTaskIsdCmd : Outport  Port=6
  WorkCmdTaskIsqCmd : Outport  Port=7
  WorkCmdTaskFreqCmd : Outport  Port=8
  SpeedCmdDir : Outport  Port=9
  wires:
  Cmd2TaskChart/8(WorkCmdTaskFreqCmd) -> WorkCmdTaskFreqCmd/1
  CurrentPolar/1 -> Isdq/7(CurrentPolar), Cmd2TaskChart/12(CurrentPolar)
  Abs/1 -> Cmd2TaskChart/11(TorqeCtrl_TorqueCmdFilterAbs)
  Cmd2TaskChart/2(WorkCmdTaskTorqueCmd) -> WorkCmdTaskTorqueCmd/1
  WorkCmdRunCmd/1 -> Cmd2TaskChart/3(WorkCmdRunCmd)
  Cmd2TaskChart/6(WorkCmdTaskIsdCmd) -> Isdq/2(TaskIsdCmd)
  SpeedCal_HighSpdZeroTrqFlg/1 -> Cmd2TaskChart/10(SpeedCal_HighSpdZeroTrqFlg)
  WorkCmdIsqCmd/1 -> Cmd2TaskChart/8(WorkCmdIsqCmd)
  Cmd2TaskChart/4(WorkCmdTaskCurrentCmd) -> WorkCmdTaskCurrentCmd/1
  WorkCmdFreqCmd/1 -> Cmd2TaskChart/9(WorkCmdFreqCmd)
  WorkCmdCurrentCmd/1 -> Cmd2TaskChart/6(WorkCmdCurrentCmd)
  WorkCmdSpeedCmd/1 -> Cmd2TaskChart/5(WorkCmdSpeedCmd)
  WorkCmdTorqueCmd/1 -> Cmd2TaskChart/4(WorkCmdTorqueCmd)
  Cmd2TaskChart/7(WorkCmdTaskIsqCmd) -> Isdq/3(TaskIsqCmd)
  WorkCmdIsdCmd/1 -> Cmd2TaskChart/1(WorkCmdIsdCmd)
  WorkState_ModeSelect/1 -> [ModeSelect], Cmd2TaskChart/2(WorkState_ModeSelect)
  WorkCmdThetaCmd/1 -> Cmd2TaskChart/7(WorkCmdThetaCmd)
  TorqeCtrl_TorqueCmdFilter/1 -> Abs/1
  Cmd2TaskChart/5(WorkCmdTaskThetaCmd) -> WorkCmdTaskThetaCmd/1
  Cmd2TaskChart/3(WorkCmdTaskSpeedCmd) -> WorkCmdTaskSpeedCmd/1
  Cmd2TaskChart/9(SpeedCmdDir) -> SpeedCmdDir/1
  Cmd2TaskChart/1(WorkCmdTaskRunCmd) -> WorkCmdTaskRunCmd/1
  [ModeSelect] -> Isdq/1(ModeSelcet)
  Isdq/1(WorkCmdTaskIsdCmd) -> WorkCmdTaskIsdCmd/1
  Isdq/2(WorkCmdTaskIsqCmd) -> WorkCmdTaskIsqCmd/1
  IdqMap_IdRef/1 -> Isdq/4(IdqMap_IdRef)
  SpeedLoopCal_PidSpdOut/1 -> Isdq/6(SpeedLoopCal_PidSpdOut)
  ParamCfgCommandSource/1 -> Isdq/8(ParamCfgCommandSource)
  IdqMap_IqRef/1 -> Isdq/5(IdqMap_IqRef)

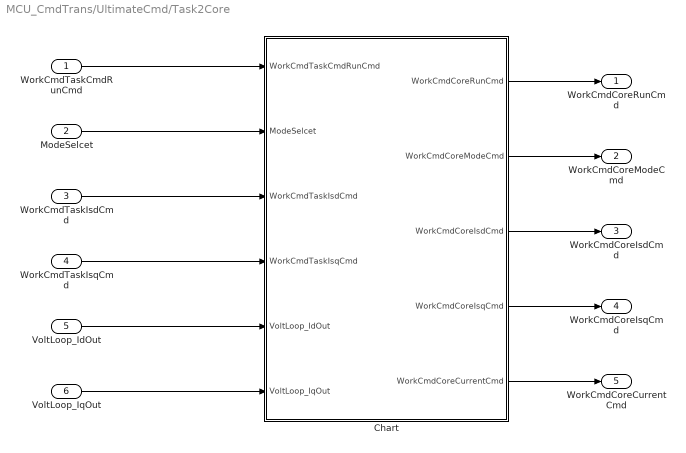
== system MCU_CmdTrans/UltimateCmd/Task2Core ==
  WorkCmdTaskCmdRunCmd : Inport
  ModeSelcet : Inport  Port=2
  WorkCmdTaskIsdCmd : Inport  Port=3
  WorkCmdTaskIsqCmd : Inport  Port=4
  VoltLoop_IdOut : Inport  Port=5
  VoltLoop_IqOut : Inport  Port=6
  Chart : Stateflow chart  TreatAsAtomicUnit=on
      settings: PortSchema="{\"entries\":[{\"content\":{\"sides\":[{\"content\":{\"connectorIds\":[\"In6\",\"In1\",\"In2\",\"In3\",\"In4\",\"In5\"]},\"type\":\"ConnectorPlacement.EquallySpacedRectSide\",\"uuid\":\"f1d33055-fd2c-400b-9297-7f9dda44e5df\"},{\"content\":{\"connectorIds\":[\"Out1\",\"Out2\",\"Out3\",\"Out4\",\"Out5\"],\"side\":\"RIGHT\"},\"type\":\"ConnectorPlacement.EquallySpacedRectSide\",\"uuid\":\"8e568ab8-3500-4880-a6e8-2ede613a6b12\"},{\"content\":{\"connectorIds\":[],\"side\":\"TOP\"},\"type\":\"ConnectorPlacement.EquallySpacedRectSide\",\"uuid\":\"7096dce0-6911-4e43-942a-ae94d3eed17e\"}]},\"type\":\"ConnectorPlacement.EquallySpacedConnector\",\"uuid\":\"bd634e07-1a6d-40e6-afbc-e5809b4cc069\"}],\"packageUris\":[\"http://schema.mathworks.com/mf0/Connector/R2020b\"],\"version\":\"1.0\"}"
  WorkCmdCoreRunCmd : Outport
  WorkCmdCoreModeCmd : Outport  Port=2
  WorkCmdCoreIsdCmd : Outport  Port=3
  WorkCmdCoreIsqCmd : Outport  Port=4
  WorkCmdCoreCurrentCmd : Outport  Port=5
  wires:
  ModeSelcet/1 -> Chart/1(ModeSelcet)
  WorkCmdTaskIsdCmd/1 -> Chart/2(WorkCmdTaskIsdCmd)
  WorkCmdTaskIsqCmd/1 -> Chart/3(WorkCmdTaskIsqCmd)
  VoltLoop_IdOut/1 -> Chart/4(VoltLoop_IdOut)
  VoltLoop_IqOut/1 -> Chart/5(VoltLoop_IqOut)
  WorkCmdTaskCmdRunCmd/1 -> Chart/6(WorkCmdTaskCmdRunCmd)
  Chart/1(WorkCmdCoreRunCmd) -> WorkCmdCoreRunCmd/1
  Chart/2(WorkCmdCoreModeCmd) -> WorkCmdCoreModeCmd/1
  Chart/3(WorkCmdCoreIsdCmd) -> WorkCmdCoreIsdCmd/1
  Chart/4(WorkCmdCoreIsqCmd) -> WorkCmdCoreIsqCmd/1
  Chart/5(WorkCmdCoreCurrentCmd) -> WorkCmdCoreCurrentCmd/1

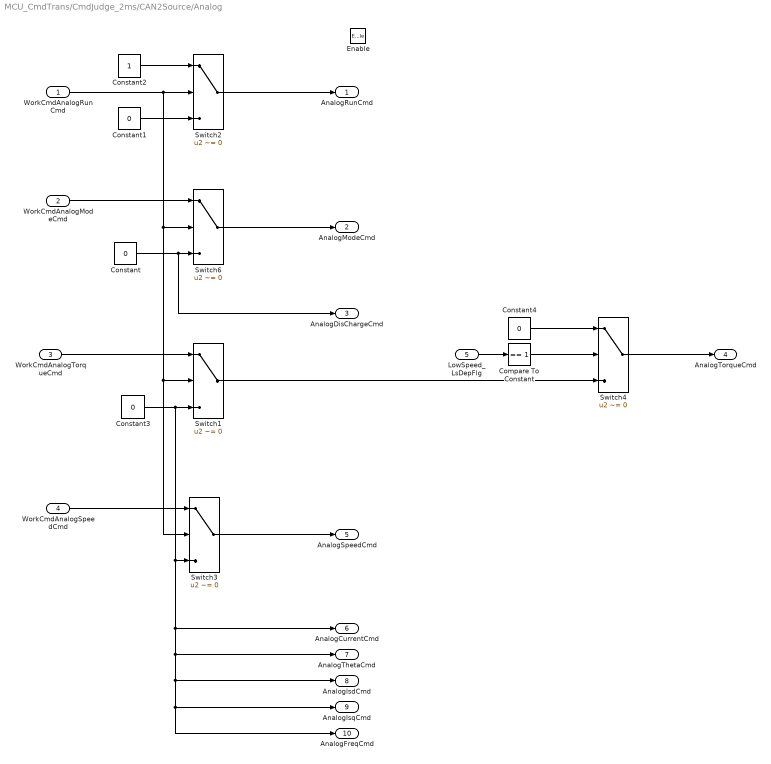
== system MCU_CmdTrans/CmdJudge_2ms/CAN2Source/Analog ==
  WorkCmdAnalogRunCmd : Inport
  WorkCmdAnalogModeCmd : Inport  Port=2
  WorkCmdAnalogTorqueCmd : Inport  Port=3
  WorkCmdAnalogSpeedCmd : Inport  Port=4
  LowSpeed_LsDepFlg : Inport  Port=5
  Enable : EnablePort
  Compare To Constant : simulink/Logic and Bit Operations/Compare To Constant  relop===  const=1  OutDataTypeStr=boolean
  Constant : Constant  Value=0  OutDataTypeStr=uint16
  Constant1 : Constant  Value=0  OutDataTypeStr=uint16
  Constant2 : Constant  OutDataTypeStr=uint16
  Constant3 : Constant  Value=0  OutDataTypeStr=single
  Constant4 : Constant  Value=0  OutDataTypeStr=single
  Switch{1..4,6} (5 alike) : Switch  Criteria=u2 ~= 0  SaturateOnIntegerOverflow=off  InputSameDT=off
  AnalogRunCmd : Outport
  AnalogModeCmd : Outport  Port=2
  AnalogDisChargeCmd : Outport  Port=3
  AnalogTorqueCmd : Outport  Port=4
  AnalogSpeedCmd : Outport  Port=5
  AnalogCurrentCmd : Outport  Port=6
  AnalogThetaCmd : Outport  Port=7
  AnalogIsdCmd : Outport  Port=8
  AnalogIsqCmd : Outport  Port=9
  AnalogFreqCmd : Outport  Port=10
  wires:
  WorkCmdAnalogRunCmd/1 -> Switch2/2, Switch3/2, Switch1/2, Switch6/2
  WorkCmdAnalogModeCmd/1 -> Switch6/1
  Switch6/1 -> AnalogModeCmd/1
  Constant/1 -> AnalogDisChargeCmd/1, Switch6/3
  Switch2/1 -> AnalogRunCmd/1
  Constant1/1 -> Switch2/3
  Constant2/1 -> Switch2/1
  WorkCmdAnalogTorqueCmd/1 -> Switch1/1
  Switch1/1 -> Switch4/3
  WorkCmdAnalogSpeedCmd/1 -> Switch3/1
  Switch3/1 -> AnalogSpeedCmd/1
  Constant3/1 -> AnalogFreqCmd/1, AnalogIsqCmd/1, AnalogIsdCmd/1, AnalogThetaCmd/1, AnalogCurrentCmd/1, Switch3/3, Switch1/3
  LowSpeed_LsDepFlg/1 -> Compare To Constant/1
  Compare To Constant/1 -> Switch4/2
  Switch4/1 -> AnalogTorqueCmd/1
  Constant4/1 -> Switch4/1

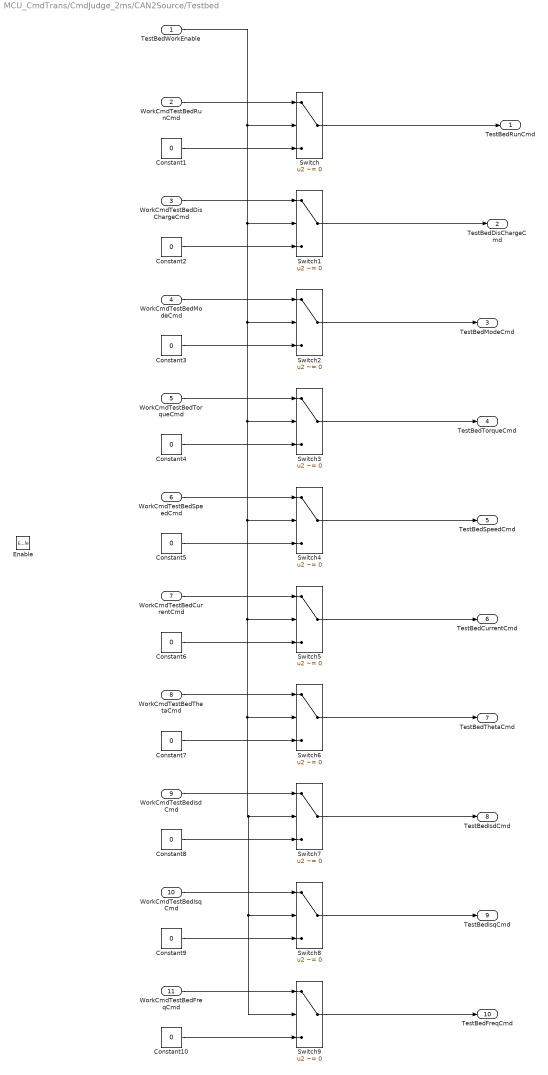
== system MCU_CmdTrans/CmdJudge_2ms/CAN2Source/Testbed ==
  TestBedWorkEnable : Inport
  WorkCmdTestBedRunCmd : Inport  Port=2
  WorkCmdTestBedDisChargeCmd : Inport  Port=3
  WorkCmdTestBedModeCmd : Inport  Port=4
  WorkCmdTestBedTorqueCmd : Inport  Port=5
  WorkCmdTestBedSpeedCmd : Inport  Port=6
  WorkCmdTestBedCurrentCmd : Inport  Port=7
  WorkCmdTestBedThetaCmd : Inport  Port=8
  WorkCmdTestBedIsdCmd : Inport  Port=9
  WorkCmdTestBedIsqCmd : Inport  Port=10
  WorkCmdTestBedFreqCmd : Inport  Port=11
  Enable : EnablePort
  Constant1 : Constant  Value=0  OutDataTypeStr=uint16
  Constant{4..10} (7 alike) : Constant  Value=0  OutDataTypeStr=single
  Constant2 : Constant  Value=0  OutDataTypeStr=uint16
  Constant3 : Constant  Value=0  OutDataTypeStr=uint16
  Switch{,1..9} (10 alike) : Switch  Criteria=u2 ~= 0  SaturateOnIntegerOverflow=off  InputSameDT=off
  TestBedRunCmd : Outport
  TestBedDisChargeCmd : Outport  Port=2
  TestBedModeCmd : Outport  Port=3
  TestBedTorqueCmd : Outport  Port=4
  TestBedSpeedCmd : Outport  Port=5
  TestBedCurrentCmd : Outport  Port=6
  TestBedThetaCmd : Outport  Port=7
  TestBedIsdCmd : Outport  Port=8
  TestBedIsqCmd : Outport  Port=9
  TestBedFreqCmd : Outport  Port=10
  wires:
  Constant1/1 -> Switch/3
  WorkCmdTestBedRunCmd/1 -> Switch/1
  WorkCmdTestBedDisChargeCmd/1 -> Switch1/1
  Constant2/1 -> Switch1/3
  WorkCmdTestBedModeCmd/1 -> Switch2/1
  Constant3/1 -> Switch2/3
  TestBedWorkEnable/1 -> Switch9/2, Switch8/2, Switch7/2, Switch6/2, Switch5/2, Switch4/2, Switch3/2, Switch2/2, Switch1/2, Switch/2
  WorkCmdTestBedTorqueCmd/1 -> Switch3/1
  Constant4/1 -> Switch3/3
  WorkCmdTestBedSpeedCmd/1 -> Switch4/1
  WorkCmdTestBedCurrentCmd/1 -> Switch5/1
  WorkCmdTestBedThetaCmd/1 -> Switch6/1
  WorkCmdTestBedIsdCmd/1 -> Switch7/1
  WorkCmdTestBedIsqCmd/1 -> Switch8/1
  WorkCmdTestBedFreqCmd/1 -> Switch9/1
  Constant5/1 -> Switch4/3
  Constant6/1 -> Switch5/3
  Constant7/1 -> Switch6/3
  Constant8/1 -> Switch7/3
  Constant9/1 -> Switch8/3
  Constant10/1 -> Switch9/3
  Switch/1 -> TestBedRunCmd/1
  Switch1/1 -> TestBedDisChargeCmd/1
  Switch2/1 -> TestBedModeCmd/1
  Switch3/1 -> TestBedTorqueCmd/1
  Switch4/1 -> TestBedSpeedCmd/1
  Switch5/1 -> TestBedCurrentCmd/1
  Switch6/1 -> TestBedThetaCmd/1
  Switch7/1 -> TestBedIsdCmd/1
  Switch8/1 -> TestBedIsqCmd/1
  Switch9/1 -> TestBedFreqCmd/1

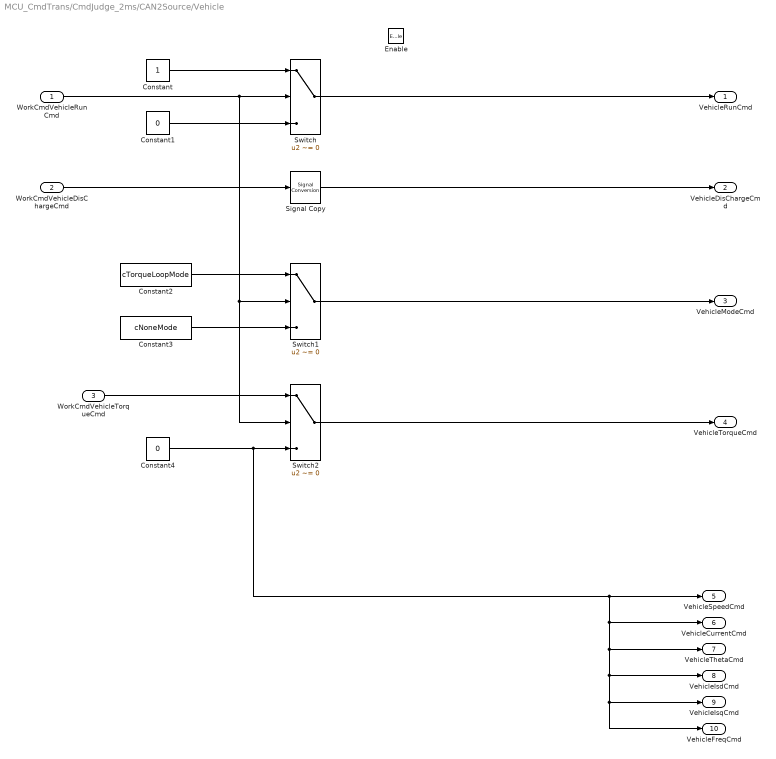
== system MCU_CmdTrans/CmdJudge_2ms/CAN2Source/Vehicle ==
  WorkCmdVehicleRunCmd : Inport
  WorkCmdVehicleDisChargeCmd : Inport  Port=2
  WorkCmdVehicleTorqueCmd : Inport  Port=3
  Enable : EnablePort
  Constant : Constant  OutDataTypeStr=uint16
  Constant1 : Constant  Value=0  OutDataTypeStr=uint16
  Constant2 : Constant  Value=cTorqueLoopMode
  Constant3 : Constant  Value=cNoneMode
  Constant4 : Constant  Value=0  OutDataTypeStr=single
  Signal Copy : SignalConversion  OverrideOpt=off
  Switch : Switch  Criteria=u2 ~= 0  SaturateOnIntegerOverflow=off  InputSameDT=off
  Switch1 : Switch  Criteria=u2 ~= 0  SaturateOnIntegerOverflow=off  InputSameDT=off
  Switch2 : Switch  Criteria=u2 ~= 0  SaturateOnIntegerOverflow=off  InputSameDT=off
  VehicleRunCmd : Outport
  VehicleDisChargeCmd : Outport  Port=2
  VehicleModeCmd : Outport  Port=3
  VehicleTorqueCmd : Outport  Port=4
  VehicleSpeedCmd : Outport  Port=5
  VehicleCurrentCmd : Outport  Port=6
  VehicleThetaCmd : Outport  Port=7
  VehicleIsdCmd : Outport  Port=8
  VehicleIsqCmd : Outport  Port=9
  VehicleFreqCmd : Outport  Port=10
  wires:
  WorkCmdVehicleRunCmd/1 -> Switch2/2, Switch1/2, Switch/2
  Constant/1 -> Switch/1
  Switch/1 -> VehicleRunCmd/1
  Constant1/1 -> Switch/3
  WorkCmdVehicleDisChargeCmd/1 -> Signal Copy/1
  Signal Copy/1 -> VehicleDisChargeCmd/1
  Constant2/1 -> Switch1/1
  Constant3/1 -> Switch1/3
  Switch1/1 -> VehicleModeCmd/1
  WorkCmdVehicleTorqueCmd/1 -> Switch2/1
  Constant4/1 -> VehicleThetaCmd/1, VehicleFreqCmd/1, VehicleIsqCmd/1, VehicleIsdCmd/1, VehicleCurrentCmd/1, VehicleSpeedCmd/1, Switch2/3
  Switch2/1 -> VehicleTorqueCmd/1
